simulink model "W2Q3"  (R2020b)
settings: Solver=VariableStepAuto  StartTime=0.0  StopTime=120  RelTol=1e-3
model workspace (MAT data in the model file):
  b = 50
  m = 1000
  u = 500
values from neighbouring files (symbols this model uses):
  Ki = 50    [variable_3.m]
  Kp = 600    [variable_3.m]
settings Model: Creator=VIVEK  LastModifiedBy=VIVEK

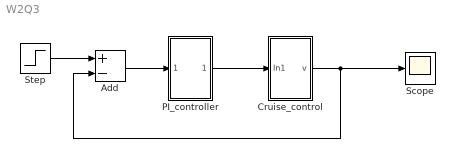
== system W2Q3 ==
  Add : Sum  Inputs=+-
  Cruise_control : Subsystem
  PI_controller : Subsystem
  Scope : Scope
  Step : Step  Time=0  After=u  SampleTime=0
  wires:
  Cruise_control/1(v) -> Add/2, Scope/1
  PI_controller/1(Out1) -> Cruise_control/1(In1)
  Step/1 -> Add/1
  Add/1 -> PI_controller/1(In1)

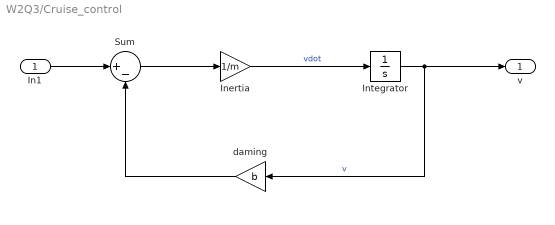
== system W2Q3/Cruise_control ==
  In1 : Inport
  Inertia : Gain  Gain=1/m
  Integrator : Integrator
  Sum : Sum  Inputs=|+-
  daming : Gain  Gain=b
  v : Outport
  wires:
  In1/1 -> Sum/1
  daming/1 -> Sum/2
  Integrator/1 -> v/1, daming/1  "v"
  Sum/1 -> Inertia/1
  Inertia/1 -> Integrator/1  "vdot"

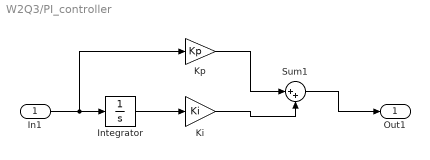
== system W2Q3/PI_controller ==
  In1 : Inport
  Integrator : Integrator
  Ki : Gain  Gain=Ki
  Kp : Gain  Gain=Kp
  Sum1 : Sum  Inputs=|++
  Out1 : Outport
  wires:
  Ki/1 -> Sum1/2
  In1/1 -> Integrator/1, Kp/1
  Integrator/1 -> Ki/1
  Sum1/1 -> Out1/1
  Kp/1 -> Sum1/1
